simulink model "goertzel_split"  (R2020b)
settings: Solver=VariableStepAuto  StartTime=0.0  StopTime=1  RelTol=1e-3
settings Model: Creator=pablo  LastModifiedBy=pablo

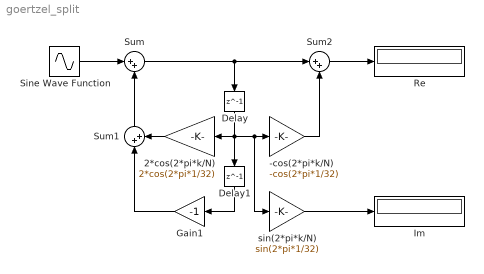
== system goertzel_split ==
  -cos(2*pi*k/N) : Gain  Gain=-cos(2*pi*1/32)
  2*cos(2*pi*k/N) : Gain  Gain=2*cos(2*pi*1/32)
  Delay : Delay  DelayLength=1  InitialCondition=0
  Delay1 : Delay  DelayLength=1  InitialCondition=0
  Gain1 : Gain  Gain=-1
  Im : Display
  Re : Display
  Sine Wave Function : Sin  SineType=Sample based  Samples=32  SampleTime=1/32
  Sum : Sum  Inputs=|++
  Sum1 : Sum  Inputs=|++
  Sum2 : Sum  Inputs=|++
  sin(2*pi*k/N) : Gain  Gain=sin(2*pi*1/32)
  wires:
  2*cos(2*pi*k/N)/1 -> Sum1/2
  Sum2/1 -> Re/1
  Sum1/1 -> Sum/2
  -cos(2*pi*k/N)/1 -> Sum2/2
  Gain1/1 -> Sum1/1
  Sine Wave Function/1 -> Sum/1
  Delay/1 -> Delay1/1, 2*cos(2*pi*k/N)/1, sin(2*pi*k/N)/1, -cos(2*pi*k/N)/1
  Sum/1 -> Sum2/1, Delay/1
  Delay1/1 -> Gain1/1
  sin(2*pi*k/N)/1 -> Im/1
